simulink model "sm"  (R2017a)
settings: Solver=FixedStepAuto  StartTime=0.0  StopTime=10.0  FixedStep=1  RelTol=1e-3
settings Model: Creator=erich  LastModifiedBy=erich

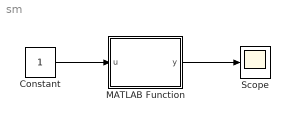
== system sm ==
  Constant : Constant
  MATLAB Function : MATLAB Function  TreatAsAtomicUnit=on
  Scope : Scope
  wires:
  Constant/1 -> MATLAB Function/1(u)
  MATLAB Function/1(y) -> Scope/1

== matlab function sm/MATLAB Function ==
  data: u input; y output; opt parameter
function y = fcn(u, opt)


H = [1 1; 1 1];
F = [1; 1];

[x] = qpOASES(H, F, [-5;-5], [5;5], opt)


y = u;
